simulink model "FinalProjectSimulation"  (R2023a)
settings: Solver=FixedStepAuto  StartTime=0.0  StopTime=t_final  FixedStep=dt  RelTol=1e-3
values from neighbouring files (symbols this model uses):
  dq_0 = [0; 0; 0]    [Initialization.m]
  dt = 1.00e-03    (= 0.001)    [Initialization.m]
  ikInitGuessSim = ikInitGuess    [defineTrajectory.m]
  P2_R2_waypoints = horzcat(initPosition,     [0.4000, 0, 0.8500 ... (first row only)    [defineTrajectory.m]
  P2_R2_waypointTimes = 0:3:6    [defineTrajectory.m]
  P2_R2_waypointVels = 0.1*[    1.5,  0,   1 ... (first row only)    [defineTrajectory.m]
  R2_T_R1 = [-1,  0,  0, P2_R1_pose(1)*2 + rod_length(1) ... (first row only)    [Initialization.m]
  rod_length = [0.20;0;0]    [Initialization.m]
  t_final = 30    [Initialization.m]
libraries: simulink x14, robotcorelib x6, robotmaniplib x1
settings Model: Creator=lukasz  LastModifiedBy=lukasz
settings OptimizationCC: ReuseModelBlockBuffer=off

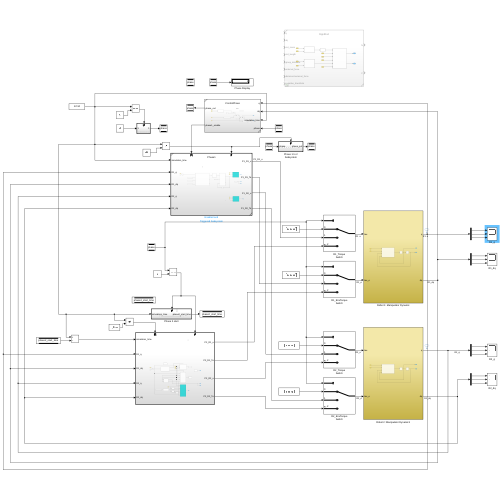
[thumbnail: Simulink's stored preview of the top-level diagram]
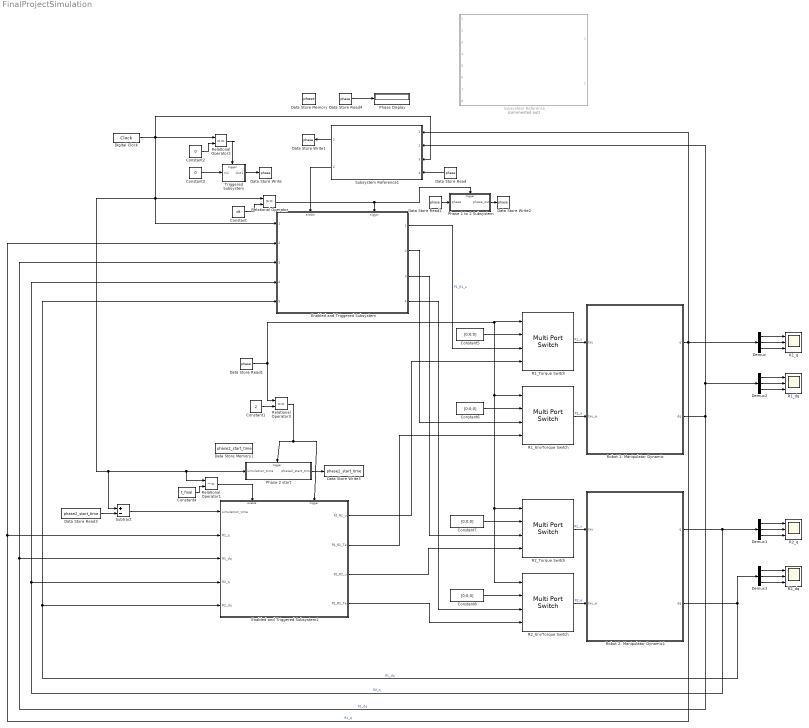
== system FinalProjectSimulation ==
  Constant : Constant  Value=dt
  Constant1 : Constant  Value=2
  Constant2 : Constant  Value=0
  Constant3 : Constant  Value=0  OutDataTypeStr=uint8
  Constant4 : Constant  Value=t_final
  Constant{5..8} (4 alike) : Constant  Value=[0;0;0]
  Data Store Memory : DataStoreMemory  DataStoreName=phase  WriteAfterWriteMsg=warning  ShowAdditionalParam=off  OutDataTypeStr=uint8
  Data Store Memory1 : DataStoreMemory  DataStoreName=phase2_start_time  WriteAfterWriteMsg=warning  InitialValue=-inf  ShowAdditionalParam=off
  Data Store Read{,1..2,4} (4 alike) : DataStoreRead  DataStoreName=phase  IndexOptions=Index vector (dialog)  Indices=1  OutputSizes=1
  Data Store Read3 : DataStoreRead  DataStoreName=phase2_start_time  IndexOptions=Index vector (dialog)  Indices=1  OutputSizes=1
  Data Store Write : DataStoreWrite  DataStoreName=phase  IndexOptions=Index vector (dialog)  Indices=1  OutputSizes=1
  Data Store Write1 : DataStoreWrite  DataStoreName=phase  IndexOptions=Index vector (dialog)  Indices=1  OutputSizes=1
  Data Store Write2 : DataStoreWrite  DataStoreName=phase  IndexOptions=Index vector (dialog)  Indices=1  OutputSizes=1
  Data Store Write3 : DataStoreWrite  DataStoreName=phase2_start_time  IndexOptions=Index vector (dialog)  Indices=1  OutputSizes=1
  Demux{,1..3} (4 alike) : Demux  Outputs=3
  Digital Clock : DigitalClock  SampleTime=dt
  Enabled and Triggered Subsystem : Subsystem  TreatAsAtomicUnit=on  ReferencedSubsystem=Phase1
  Enabled and Triggered Subsystem2 : Subsystem  TreatAsAtomicUnit=on
  Phase 1 to 2 Subsystem : Subsystem  TreatAsAtomicUnit=on
  Phase 2 start : Subsystem  TreatAsAtomicUnit=on
  Phase Display : Display
  R1_EnvTorque Switch : MultiPortSwitch  DataPortOrder=Specify indices  DataPortIndices={0,1,2}  SaturateOnIntegerOverflow=off  InputSameDT=off
  R1_Torque Switch : MultiPortSwitch  DataPortOrder=Specify indices  DataPortIndices={0,1,2}  SaturateOnIntegerOverflow=off  InputSameDT=off
  R1_dq : Scope  NumInputPorts=3
  R1_q : Scope  NumInputPorts=3
  R2_EnvTorque Switch : MultiPortSwitch  DataPortOrder=Specify indices  DataPortIndices={0,1,2}  SaturateOnIntegerOverflow=off  InputSameDT=off
  R2_Torque Switch : MultiPortSwitch  DataPortOrder=Specify indices  DataPortIndices={0,1,2}  SaturateOnIntegerOverflow=off  InputSameDT=off
  R2_dq : Scope  NumInputPorts=3
  R2_q : Scope  NumInputPorts=3
  Relational Operator : RelationalOperator  OutDataTypeStr=boolean  RndMeth=Simplest  InputSameDT=off
  Relational Operator1 : RelationalOperator  Operator=~=  OutDataTypeStr=boolean  RndMeth=Simplest  InputSameDT=off
  Relational Operator2 : RelationalOperator  Operator===  OutDataTypeStr=boolean  RndMeth=Simplest  InputSameDT=off
  Relational Operator3 : RelationalOperator  Operator===  OutDataTypeStr=boolean  RndMeth=Simplest  InputSameDT=off
  Robot 1: Manipulator Dynamic : Subsystem
  Robot 2: Manipulator Dynamic1 : Subsystem
  Subsystem Reference : Subsystem  Commented=on  ReferencedSubsystem=RigidRod
  Subsystem Reference1 : Subsystem  ReferencedSubsystem=ControlPhase
  Subtract : Sum  Inputs=+-
  Triggered Subsystem : Subsystem  TreatAsAtomicUnit=on
  wires:
  Demux/1 -> R1_q/1
  Demux/2 -> R1_q/2
  Demux/3 -> R1_q/3
  Constant/1 -> Relational Operator/2
  Relational Operator/1 -> Phase 1 to 2 Subsystem/Trigger, Enabled and Triggered Subsystem/Trigger
  Enabled and Triggered Subsystem/1 -> R1_Torque Switch/3  "P1_R1_u"
  R1_Torque Switch/1 -> Robot 1: Manipulator Dynamic/1(tau)  "R1_u"
  Robot 1: Manipulator Dynamic/2(dq) -> Subsystem Reference1/2, Demux2/1, Enabled and Triggered Subsystem/3, Enabled and Triggered Subsystem2/3(R1_dq)  "R1_dq"
  Robot 1: Manipulator Dynamic/1(q) -> Enabled and Triggered Subsystem/2, Enabled and Triggered Subsystem2/2(R1_q), Subsystem Reference1/1, Demux/1  "R1_q"
  Subsystem Reference1/2 -> Enabled and Triggered Subsystem/Enable
  Constant2/1 -> Relational Operator2/2
  Relational Operator2/1 -> Triggered Subsystem/Trigger
  Triggered Subsystem/1(Out1) -> Data Store Write/1
  Constant3/1 -> Triggered Subsystem/1(In1)
  Data Store Read/1 -> Subsystem Reference1/4
  Subsystem Reference1/1 -> Data Store Write1/1
  Data Store Read1/1 -> Relational Operator3/1, R1_Torque Switch/1, R2_EnvTorque Switch/1, R2_Torque Switch/1, R1_EnvTorque Switch/1
  Phase 1 to 2 Subsystem/1(phase_out) -> Data Store Write2/1
  Data Store Read2/1 -> Phase 1 to 2 Subsystem/1(phase)
  Constant1/1 -> Relational Operator3/2
  Relational Operator3/1 -> Enabled and Triggered Subsystem2/Trigger, Phase 2 start/Trigger
  Digital Clock/1 -> Relational Operator/1, Enabled and Triggered Subsystem/1, Relational Operator1/1, Phase 2 start/1(simulation_time), Subtract/1, Subsystem Reference1/3, Relational Operator2/1
  Data Store Read4/1 -> Phase Display/1
  Enabled and Triggered Subsystem/2 -> R1_EnvTorque Switch/3
  R1_EnvTorque Switch/1 -> Robot 1: Manipulator Dynamic/2(tau_e)  "R1_e"
  Enabled and Triggered Subsystem2/1(P2_R1_u) -> R1_Torque Switch/4
  Enabled and Triggered Subsystem2/2(P2_R1_Te) -> R1_EnvTorque Switch/4
  Phase 2 start/1(phase2_start_time) -> Data Store Write3/1
  Subtract/1 -> Enabled and Triggered Subsystem2/1(simulation_time)
  Data Store Read3/1 -> Subtract/2
  Relational Operator1/1 -> Enabled and Triggered Subsystem2/Enable
  Constant4/1 -> Relational Operator1/2
  R2_EnvTorque Switch/1 -> Robot 2: Manipulator Dynamic1/2(tau_e)  "R2_e"
  R2_Torque Switch/1 -> Robot 2: Manipulator Dynamic1/1(tau)  "R2_u"
  Demux1/3 -> R2_q/3
  Robot 2: Manipulator Dynamic1/1(q) -> Enabled and Triggered Subsystem/4, Enabled and Triggered Subsystem2/4(R2_q), Demux1/1  "R2_q"
  Demux1/1 -> R2_q/1
  Demux1/2 -> R2_q/2
  Enabled and Triggered Subsystem2/3(P2_R2_u) -> R2_Torque Switch/4
  Enabled and Triggered Subsystem2/4(P2_R2_Te) -> R2_EnvTorque Switch/4
  Enabled and Triggered Subsystem/3 -> R2_Torque Switch/3
  Enabled and Triggered Subsystem/4 -> R2_EnvTorque Switch/3
  Robot 2: Manipulator Dynamic1/2(dq) -> Enabled and Triggered Subsystem/5, Enabled and Triggered Subsystem2/5(R2_dq), Demux3/1  "R1_dq"
  Constant5/1 -> R1_Torque Switch/2
  Constant6/1 -> R1_EnvTorque Switch/2
  Constant7/1 -> R2_Torque Switch/2
  Constant8/1 -> R2_EnvTorque Switch/2
  Demux2/3 -> R1_dq/3
  Demux2/1 -> R1_dq/1
  Demux2/2 -> R1_dq/2
  Demux3/3 -> R2_dq/3
  Demux3/2 -> R2_dq/2
  Demux3/1 -> R2_dq/1

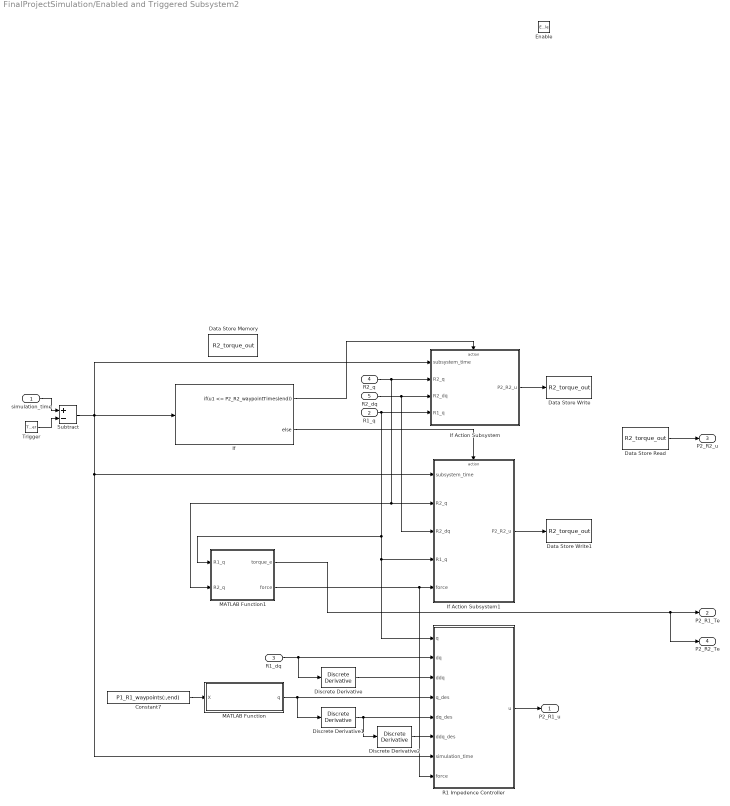
== system FinalProjectSimulation/Enabled and Triggered Subsystem2 ==
  simulation_time : Inport
  R1_q : Inport  Port=2
  R1_dq : Inport  Port=3
  R2_q : Inport  Port=4
  R2_dq : Inport  Port=5
  Enable : EnablePort
  Trigger : TriggerPort  VariantControl=(inherit)  ShowOutputPort=on
  Constant7 : Constant  Value=P1_R1_waypoints(:,end)  VectorParams1D=off  SampleTime=-1
  Data Store Memory : DataStoreMemory  DataStoreName=R2_torque_out  WriteAfterWriteMsg=warning  InitialValue=[0;0;0]  ShowAdditionalParam=off  Dimensions=3
  Data Store Read : DataStoreRead  DataStoreName=R2_torque_out  IndexOptions=Index vector (dialog)  Indices=1  OutputSizes=1
  Data Store Write : DataStoreWrite  DataStoreName=R2_torque_out  IndexOptions=Index vector (dialog)  Indices=1  OutputSizes=1
  Data Store Write1 : DataStoreWrite  DataStoreName=R2_torque_out  IndexOptions=Index vector (dialog)  Indices=1  OutputSizes=1
  Discrete Derivative : simulink/Discrete/Discrete Derivative  gainval=1.0  ICPrevScaledInput=1  OutMin=[]  OutMax=[]  OutDataType=fixdt(1, 16)  OutScaling=2^-10  DoSatur=off
  Discrete Derivative1 : simulink/Discrete/Discrete Derivative  gainval=1.0  ICPrevScaledInput=1  OutMin=[]  OutMax=[]  OutDataType=fixdt(1, 16)  OutScaling=2^-10  DoSatur=off
  Discrete Derivative2 : simulink/Discrete/Discrete Derivative  gainval=1.0  ICPrevScaledInput=1  OutMin=[]  OutMax=[]  OutDataType=fixdt(1, 16)  OutScaling=2^-10  DoSatur=off
  If : If  IfExpression=u1 <= P2_R2_waypointTimes(end)
  If Action Subsystem : Subsystem  TreatAsAtomicUnit=on
  If Action Subsystem1 : Subsystem  TreatAsAtomicUnit=on
  MATLAB Function : MATLAB Function  TreatAsAtomicUnit=on
  MATLAB Function1 : MATLAB Function  TreatAsAtomicUnit=on
  R1 Impedence Controller : Subsystem
  Subtract : Sum  Inputs=+-
  P2_R1_u : Outport
  P2_R1_Te : Outport  Port=2
  P2_R2_u : Outport  Port=3
  P2_R2_Te : Outport  Port=4
  wires:
  R2_dq/1 -> If Action Subsystem1/3(R2_dq), If Action Subsystem/3(R2_dq)
  R1 Impedence Controller/1(u) -> P2_R1_u/1
  Trigger/1 -> Subtract/2
  R2_q/1 -> MATLAB Function1/2(R2_q), If Action Subsystem1/2(R2_q), If Action Subsystem/2(R2_q)
  simulation_time/1 -> Subtract/1
  MATLAB Function1/1(torque_e) -> P2_R2_Te/1, P2_R1_Te/1
  R1_dq/1 -> Discrete Derivative/1, R1 Impedence Controller/2(dq)
  Constant7/1 -> MATLAB Function/1(X)
  MATLAB Function/1(q) -> Discrete Derivative1/1, R1 Impedence Controller/4(q_des)
  If/1 -> If Action Subsystem/Action
  Subtract/1 -> If/1, If Action Subsystem/1(subsystem_time), R1 Impedence Controller/7(simulation_time), If Action Subsystem1/1(subsystem_time)
  If Action Subsystem/1(P2_R2_u) -> Data Store Write/1
  Data Store Read/1 -> P2_R2_u/1
  If/2 -> If Action Subsystem1/Action
  If Action Subsystem1/1(P2_R2_u) -> Data Store Write1/1
  R1_q/1 -> If Action Subsystem/4(R1_q), If Action Subsystem1/4(R1_q), R1 Impedence Controller/1(q), MATLAB Function1/1(R1_q)
  Discrete Derivative/1 -> R1 Impedence Controller/3(ddq)
  Discrete Derivative1/1 -> Discrete Derivative2/1, R1 Impedence Controller/5(dq_des)
  Discrete Derivative2/1 -> R1 Impedence Controller/6(ddq_des)
  MATLAB Function1/2(force) -> R1 Impedence Controller/8(force), If Action Subsystem1/5(force)

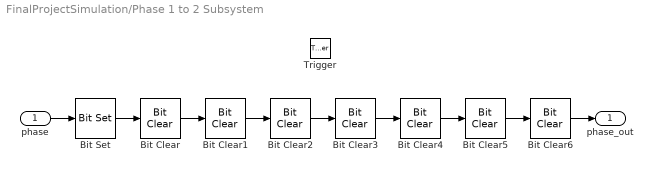
== system FinalProjectSimulation/Phase 1 to 2 Subsystem ==
  phase : Inport
  Trigger : TriggerPort  VariantControl=(inherit)
  Bit Clear : simulink/Logic and Bit Operations/Bit Clear  iBit=1
  Bit Clear1 : simulink/Logic and Bit Operations/Bit Clear  iBit=2
  Bit Clear2 : simulink/Logic and Bit Operations/Bit Clear  iBit=3
  Bit Clear3 : simulink/Logic and Bit Operations/Bit Clear  iBit=4
  Bit Clear4 : simulink/Logic and Bit Operations/Bit Clear  iBit=5
  Bit Clear5 : simulink/Logic and Bit Operations/Bit Clear  iBit=6
  Bit Clear6 : simulink/Logic and Bit Operations/Bit Clear  iBit=7
  Bit Set : simulink/Logic and Bit Operations/Bit Set  iBit=0
  phase_out : Outport
  wires:
  Bit Clear6/1 -> phase_out/1
  Bit Clear5/1 -> Bit Clear6/1
  Bit Clear4/1 -> Bit Clear5/1
  Bit Clear3/1 -> Bit Clear4/1
  Bit Clear2/1 -> Bit Clear3/1
  Bit Clear1/1 -> Bit Clear2/1
  Bit Clear/1 -> Bit Clear1/1
  phase/1 -> Bit Set/1
  Bit Set/1 -> Bit Clear/1

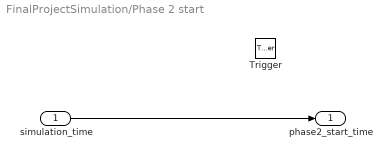
== system FinalProjectSimulation/Phase 2 start ==
  simulation_time : Inport
  Trigger : TriggerPort  VariantControl=(inherit)
  phase2_start_time : Outport
  wires:
  simulation_time/1 -> phase2_start_time/1

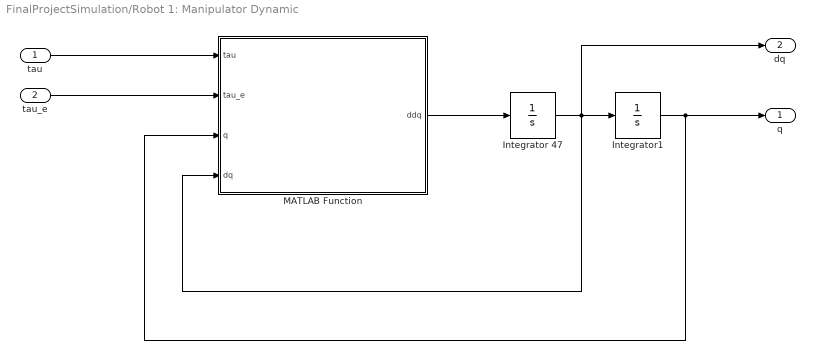
== system FinalProjectSimulation/Robot 1: Manipulator Dynamic ==
  tau : Inport
  tau_e : Inport  Port=2
  Integrator 47 : Integrator  InitialCondition=dq_0
  Integrator1 : Integrator  InitialCondition=ikInitGuessSim
  MATLAB Function : MATLAB Function  TreatAsAtomicUnit=on
  q : Outport
  dq : Outport  Port=2
  wires:
  MATLAB Function/1(ddq) -> Integrator 47/1
  tau/1 -> MATLAB Function/1(tau)
  tau_e/1 -> MATLAB Function/2(tau_e)
  Integrator1/1 -> q/1, MATLAB Function/3(q)
  Integrator 47/1 -> dq/1, MATLAB Function/4(dq), Integrator1/1

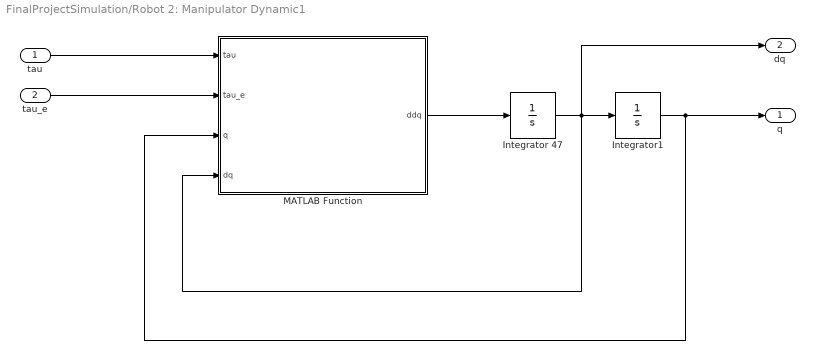
== system FinalProjectSimulation/Robot 2: Manipulator Dynamic1 ==
  tau : Inport
  tau_e : Inport  Port=2
  Integrator 47 : Integrator  InitialCondition=dq_0
  Integrator1 : Integrator  InitialCondition=ikInitGuessSim
  MATLAB Function : MATLAB Function  TreatAsAtomicUnit=on
  q : Outport
  dq : Outport  Port=2
  wires:
  MATLAB Function/1(ddq) -> Integrator 47/1
  tau/1 -> MATLAB Function/1(tau)
  tau_e/1 -> MATLAB Function/2(tau_e)
  Integrator1/1 -> q/1, MATLAB Function/3(q)
  Integrator 47/1 -> dq/1, MATLAB Function/4(dq), Integrator1/1

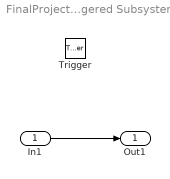
== system FinalProjectSimulation/Triggered Subsystem ==
  In1 : Inport
  Trigger : TriggerPort  VariantControl=(inherit)
  Out1 : Outport
  wires:
  In1/1 -> Out1/1

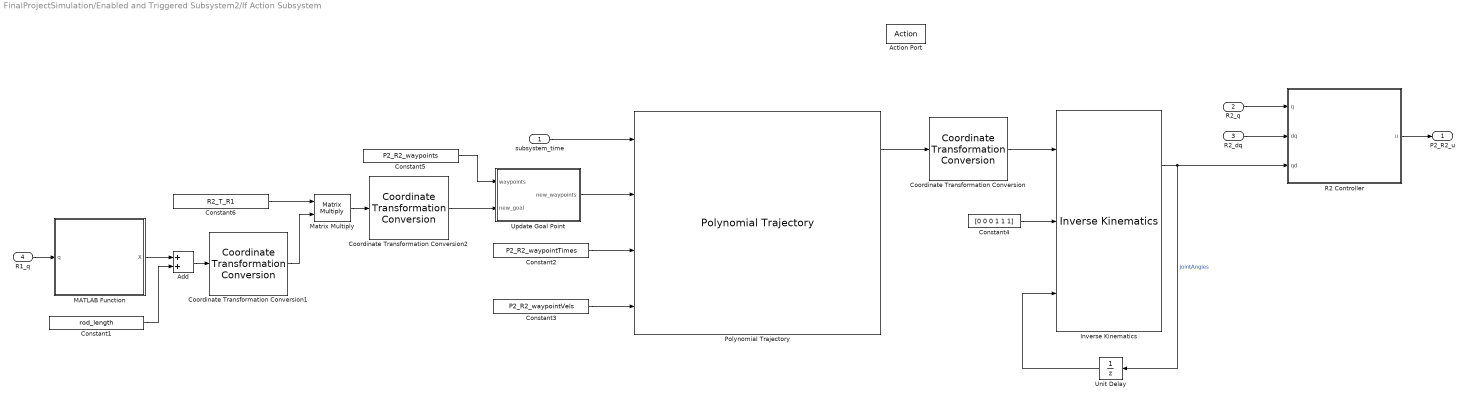
== system FinalProjectSimulation/Enabled and Triggered Subsystem2/If Action Subsystem ==
  subsystem_time : Inport
  R2_q : Inport  Port=2
  R2_dq : Inport  Port=3
  R1_q : Inport  Port=4
  Action Port : ActionPort  ActionPortLabel=if(u1 <= P2_R2_waypointTimes(end))
  Add : Sum
  Constant1 : Constant  Value=rod_length  VectorParams1D=off  SampleTime=-1
  Constant2 : Constant  Value=P2_R2_waypointTimes  VectorParams1D=off  SampleTime=-1
  Constant3 : Constant  Value=P2_R2_waypointVels  VectorParams1D=off  SampleTime=-1
  Constant4 : Constant  Value=[0 0 0 1 1 1]  VectorParams1D=off
  Constant5 : Constant  Value=P2_R2_waypoints  VectorParams1D=off  SampleTime=-1
  Constant6 : Constant  Value=R2_T_R1  VectorParams1D=off  SampleTime=-1
  Coordinate Transformation Conversion : robotcorelib/Coordinate Transformation Conversion  InputRepresentation=Translation Vector  InputEulerSequence=ZYX  ShowTrVecInputPort=on  OutputRepresentation=Homogeneous Transformation  OutputEulerSequence=ZYX  ShowTrVecOutputPort=on  SimulateUsing=Code generation
  Coordinate Transformation Conversion1 : robotcorelib/Coordinate Transformation Conversion  InputRepresentation=Translation Vector  InputEulerSequence=ZYX  ShowTrVecInputPort=on  OutputRepresentation=Homogeneous Transformation  OutputEulerSequence=ZYX  ShowTrVecOutputPort=on  SimulateUsing=Code generation
  Coordinate Transformation Conversion2 : robotcorelib/Coordinate Transformation Conversion  InputRepresentation=Homogeneous Transformation  InputEulerSequence=ZYX  ShowTrVecInputPort=on  OutputRepresentation=Translation Vector  OutputEulerSequence=ZYX  ShowTrVecOutputPort=on  SimulateUsing=Code generation
  Inverse Kinematics : robotmaniplib/Inverse Kinematics  RigidBodyTree=robot1  EndEffector=Link_EE  ShowInfo=on  SolverName=BFGS Gradient Projection  EnforceJointLimits=on  MaxIterations=1500  MaxTime=10  GradientTolerance=1e-7  SolutionTolerance=1e-6  StepTolerance=1e-14  ErrorChangeTolerance=1e-12  UseErrorDamping=on  DampingBias=0.0025  SimulateUsing=Code generation
  MATLAB Function : MATLAB Function  TreatAsAtomicUnit=on
  Matrix Multiply : Product  Multiplication=Matrix(*)  RndMeth=Round
  Polynomial Trajectory : robotcorelib/Polynomial Trajectory  WaypointSource=External  Waypoints=[ 0, 2, 1, 5, 0; -1, 3, 1, 4, 4 ]  TimePoints=[ 0, 1, 2, 3, 4 ]  TimeInterval=[ 1, 4 ]  Method=Cubic Polynomial  ParameterSource=External  VelocityBoundaryCondition=zeros( 2, 5 )  AccelerationBoundaryCondition=zeros( 2, 5 )  SimulateUsing=Interpreted execution
  R2 Controller : Subsystem
  Unit Delay : UnitDelay  InitialCondition=ikInitGuessSim  SampleTime=-1  HasFrameUpgradeWarning=on
  Update Goal Point : MATLAB Function  TreatAsAtomicUnit=on
  P2_R2_u : Outport
  wires:
  Update Goal Point/1(new_waypoints) -> Polynomial Trajectory/2
  Inverse Kinematics/1 -> R2 Controller/3(qd), Unit Delay/1  "jointAngles"
  Unit Delay/1 -> Inverse Kinematics/3
  subsystem_time/1 -> Polynomial Trajectory/1
  Constant3/1 -> Polynomial Trajectory/4
  Coordinate Transformation Conversion/1 -> Inverse Kinematics/1
  Constant4/1 -> Inverse Kinematics/2
  Polynomial Trajectory/1 -> Coordinate Transformation Conversion/1
  Constant2/1 -> Polynomial Trajectory/3
  R2_dq/1 -> R2 Controller/2(dq)
  R2_q/1 -> R2 Controller/1(q)
  R2 Controller/1(u) -> P2_R2_u/1
  R1_q/1 -> MATLAB Function/1(q)
  Coordinate Transformation Conversion2/1 -> Update Goal Point/2(new_goal)
  Constant5/1 -> Update Goal Point/1(waypoints)
  MATLAB Function/1(X) -> Add/1
  Add/1 -> Coordinate Transformation Conversion1/1
  Coordinate Transformation Conversion1/1 -> Matrix Multiply/2
  Matrix Multiply/1 -> Coordinate Transformation Conversion2/1
  Constant6/1 -> Matrix Multiply/1
  Constant1/1 -> Add/2

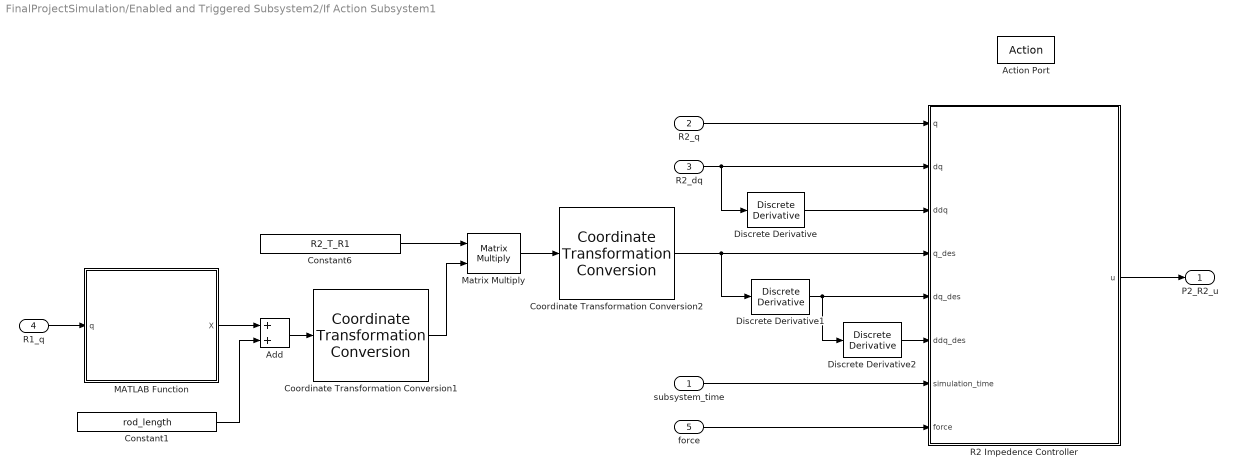
== system FinalProjectSimulation/Enabled and Triggered Subsystem2/If Action Subsystem1 ==
  subsystem_time : Inport
  R2_q : Inport  Port=2
  R2_dq : Inport  Port=3
  R1_q : Inport  Port=4
  force : Inport  Port=5
  Action Port : ActionPort  ActionPortLabel=else
  Add : Sum
  Constant1 : Constant  Value=rod_length  VectorParams1D=off  SampleTime=-1
  Constant6 : Constant  Value=R2_T_R1  VectorParams1D=off  SampleTime=-1
  Coordinate Transformation Conversion1 : robotcorelib/Coordinate Transformation Conversion  InputRepresentation=Translation Vector  InputEulerSequence=ZYX  ShowTrVecInputPort=on  OutputRepresentation=Homogeneous Transformation  OutputEulerSequence=ZYX  ShowTrVecOutputPort=on  SimulateUsing=Code generation
  Coordinate Transformation Conversion2 : robotcorelib/Coordinate Transformation Conversion  InputRepresentation=Homogeneous Transformation  InputEulerSequence=ZYX  ShowTrVecInputPort=on  OutputRepresentation=Translation Vector  OutputEulerSequence=ZYX  ShowTrVecOutputPort=on  SimulateUsing=Code generation
  Discrete Derivative : simulink/Discrete/Discrete Derivative  gainval=1.0  ICPrevScaledInput=1  OutMin=[]  OutMax=[]  OutDataType=fixdt(1, 16)  OutScaling=2^-10  DoSatur=off
  Discrete Derivative1 : simulink/Discrete/Discrete Derivative  gainval=1.0  ICPrevScaledInput=1  OutMin=[]  OutMax=[]  OutDataType=fixdt(1, 16)  OutScaling=2^-10  DoSatur=off
  Discrete Derivative2 : simulink/Discrete/Discrete Derivative  gainval=1.0  ICPrevScaledInput=1  OutMin=[]  OutMax=[]  OutDataType=fixdt(1, 16)  OutScaling=2^-10  DoSatur=off
  MATLAB Function : MATLAB Function  TreatAsAtomicUnit=on
  Matrix Multiply : Product  Multiplication=Matrix(*)  RndMeth=Round
  R2 Impedence Controller : Subsystem
  P2_R2_u : Outport
  wires:
  R2 Impedence Controller/1(u) -> P2_R2_u/1
  R2_dq/1 -> Discrete Derivative/1, R2 Impedence Controller/2(dq)
  R2_q/1 -> R2 Impedence Controller/1(q)
  subsystem_time/1 -> R2 Impedence Controller/7(simulation_time)
  R1_q/1 -> MATLAB Function/1(q)
  Coordinate Transformation Conversion1/1 -> Matrix Multiply/2
  Add/1 -> Coordinate Transformation Conversion1/1
  Constant1/1 -> Add/2
  MATLAB Function/1(X) -> Add/1
  Constant6/1 -> Matrix Multiply/1
  Matrix Multiply/1 -> Coordinate Transformation Conversion2/1
  Coordinate Transformation Conversion2/1 -> Discrete Derivative1/1, R2 Impedence Controller/4(q_des)
  Discrete Derivative/1 -> R2 Impedence Controller/3(ddq)
  Discrete Derivative1/1 -> Discrete Derivative2/1, R2 Impedence Controller/5(dq_des)
  Discrete Derivative2/1 -> R2 Impedence Controller/6(ddq_des)
  force/1 -> R2 Impedence Controller/8(force)

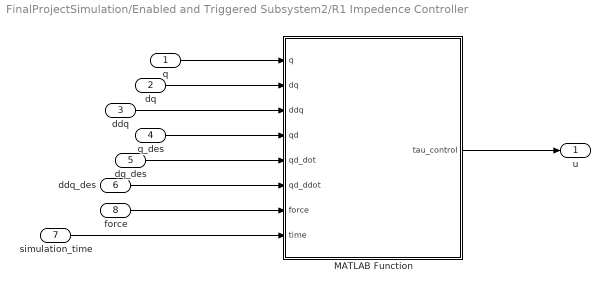
== system FinalProjectSimulation/Enabled and Triggered Subsystem2/R1 Impedence Controller ==
  q : Inport
  dq : Inport  Port=2
  ddq : Inport  Port=3
  q_des : Inport  Port=4
  dq_des : Inport  Port=5
  ddq_des : Inport  Port=6
  simulation_time : Inport  Port=7
  force : Inport  Port=8
  MATLAB Function : MATLAB Function  TreatAsAtomicUnit=on
  u : Outport
  wires:
  dq/1 -> MATLAB Function/2(dq)
  MATLAB Function/1(tau_control) -> u/1
  q_des/1 -> MATLAB Function/4(qd)
  q/1 -> MATLAB Function/1(q)
  ddq_des/1 -> MATLAB Function/6(qd_ddot)
  dq_des/1 -> MATLAB Function/5(qd_dot)
  simulation_time/1 -> MATLAB Function/8(time)
  ddq/1 -> MATLAB Function/3(ddq)
  force/1 -> MATLAB Function/7(force)

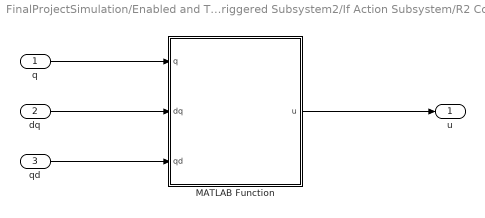
== system FinalProjectSimulation/Enabled and Triggered Subsystem2/If Action Subsystem/R2 Controller ==
  q : Inport
  dq : Inport  Port=2
  qd : Inport  Port=3
  MATLAB Function : MATLAB Function  TreatAsAtomicUnit=on
  u : Outport
  wires:
  q/1 -> MATLAB Function/1(q)
  qd/1 -> MATLAB Function/3(qd)
  MATLAB Function/1(u) -> u/1
  dq/1 -> MATLAB Function/2(dq)

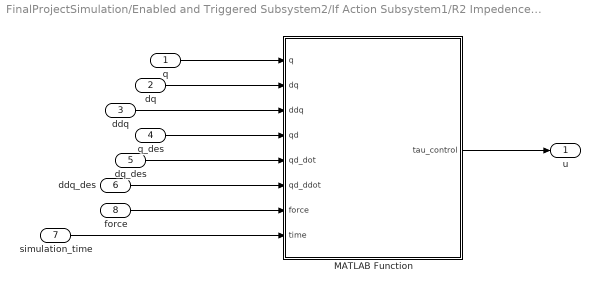
== system FinalProjectSimulation/Enabled and Triggered Subsystem2/If Action Subsystem1/R2 Impedence Controller ==
  q : Inport
  dq : Inport  Port=2
  ddq : Inport  Port=3
  q_des : Inport  Port=4
  dq_des : Inport  Port=5
  ddq_des : Inport  Port=6
  simulation_time : Inport  Port=7
  force : Inport  Port=8
  MATLAB Function : MATLAB Function  TreatAsAtomicUnit=on
  u : Outport
  wires:
  dq/1 -> MATLAB Function/2(dq)
  MATLAB Function/1(tau_control) -> u/1
  q_des/1 -> MATLAB Function/4(qd)
  q/1 -> MATLAB Function/1(q)
  ddq_des/1 -> MATLAB Function/6(qd_ddot)
  dq_des/1 -> MATLAB Function/5(qd_dot)
  simulation_time/1 -> MATLAB Function/8(time)
  ddq/1 -> MATLAB Function/3(ddq)
  force/1 -> MATLAB Function/7(force)

== matlab function FinalProjectSimulation/Enabled and Triggered Subsystem2/If Action Subsystem1/MATLAB Function ==
  data: q input; X output
function X = FWDKinematics(q)
%%% Forward Kinematic Function


%% Joint Space variables
% q is 3*1 vector of joint variables (radian), q = [q1;q2;q3]
q1 = q(1);
q2 = q(2);
q3 = q(3);

%% general physical parameters
l1 = 0.6731;
l2 = 0.432;
l3 = 0.434;
lc2 = 0.216;
lc3 = 0.164;

%% Forward Kinematic
% X is 3*1 vecto of end-effector position in task space, X = [x;y;z]

x = cos(q1) * (l2 * cos(q2) + l3 * sin(q2 + q3));
y = sin(q1) * (l2 * cos(q2) + l3 * sin(q2 + q3));
z = l1 - l2 * sin(q2) + l3 * cos(q2 + q3);

X = [x;y;z]

== matlab function FinalProjectSimulation/Enabled and Triggered Subsystem2/MATLAB Function1 ==
  data: R1_q input; torque_e output; R2_q input; force output
function [torque_e, force] = fcn(R1_q, R2_q)

k = [1, 0, 0;
      0, 1, 0;
      0, 0, 1];
comp = [0;0;0];
force = k * comp;
torque_e = [0;0;0];

== matlab function FinalProjectSimulation/Robot 1: Manipulator Dynamic/MATLAB Function ==
  data: tau input; tau_e input; q input; ddq output; dq input
function ddq = DynamicModel( tau, tau_e, q, dq)
%%%%%
% 3-DOF Puma-560 Dynamic Model Function
% H(q)* ddq + C(q) * dq + G = tau + tau_e
% q is 3*1 vector of joint variables (radian)
% H(q) is the inertia matrix
% C(q) is the matrix of Coriolis and centrifugal forces
% G(q) is  the vector of potential forces Parameters
% tau is control torque 
% tau_e is the external torque due to the interaction with the environment
%%%%%

%% Joint Space variables

q1 = q(1);
q2 = q(2);
q3 = q(3);

dq1 = dq(1);
dq2 = dq(2);
dq3 = dq(3);

%% general physical parameters

l1 = 0.6731;
l2 = 0.432;
l3 = 0.434;
lc2 = 0.216;
lc3 = 0.164;
m2 = 15.46;
m3 = 9.55;
J = 0.302;

%% Inertia Matrix Parameters

J1 = m3 * lc3^2;
J12 = (m2 * lc2^2) + (m3 * l2^2);
J13 = l2 * lc3 * m3;


h11 = J + J1 * (sin(q2 + q3))^2 + J12 * (cos(q2))^2 + 2 * J13 * cos(q2) * sin(q2+q3);
h22 = J1 + J12 + 2 * J13 * sin(q3);
h23 = J1 + J13 * sin(q3);
h32 = h23;
h33 = J1;

H = [h11, 0 ,0 ;
    0 , h22, h23;
    0 , h32, h33];

%% Coriolis Matrix Parameters

c12_1 = J1 * sin(2 * (q1 + q2)) - J12 * sin(2 * q2) + 2 * J13 * cos(2 * q2 +q3);
c13_1 = J1 * sin(2 * (q2 + q3)) + 2 * J13 * cos(q2) * cos(q2 + q3);
c11_2 = (1/2) * (-J1 * sin(2 * (q2 + q3)) + J12 * sin(2 * q2) - 2 * J13 * cos(2 * q2 + q3));
c22_2 = 2 * J13 * cos(q3);
c23_2 = J13 * cos(q3);
c22_3 = -J13 * cos(q3) * dq2;
c11_3 = (-1/2) * (J1 * sin(2 * (q2 + q3)) + J13 * cos(q2) * cos(q2 + q3));

C = [0, c12_1 * dq1, c13_1 * dq3;
    c11_2 * dq1, 0 , c22_2 * dq2 + c23_2 * dq3;
    c11_3 * dq1, c22_3 * dq2, 0];

%% Vector of Potential Forces Parameters

g = 9.81;

g21 = -g * (lc3 * m3 * sin(q2 + q3) + lc2 * m2 * cos(q2) + l2 * m3 * cos(q2));
g31 = -g * (lc3 * m3 * sin(q2 + q3));

G = [0;
    g21;
    g31];

%% Function output

ddq = inv(H)*(tau + tau_e - C * dq - G);

== matlab function FinalProjectSimulation/Robot 2: Manipulator Dynamic1/MATLAB Function ==
  data: tau input; tau_e input; q input; ddq output; dq input
function ddq = DynamicModel( tau, tau_e, q, dq)
%%%%%
% 3-DOF Puma-560 Dynamic Model Function
% H(q)* ddq + C(q) * dq + G = tau + tau_e
% q is 3*1 vector of joint variables (radian)
% H(q) is the inertia matrix
% C(q) is the matrix of Coriolis and centrifugal forces
% G(q) is  the vector of potential forces Parameters
% tau is control torque 
% tau_e is the external torque due to the interaction with the environment
%%%%%

%% Joint Space variables

q1 = q(1);
q2 = q(2);
q3 = q(3);

dq1 = dq(1);
dq2 = dq(2);
dq3 = dq(3);

%% general physical parameters

l1 = 0.6731;
l2 = 0.432;
l3 = 0.434;
lc2 = 0.216;
lc3 = 0.164;
m2 = 15.46;
m3 = 9.55;
J = 0.302;

%% Inertia Matrix Parameters

J1 = m3 * lc3^2;
J12 = (m2 * lc2^2) + (m3 * l2^2);
J13 = l2 * lc3 * m3;


h11 = J + J1 * (sin(q2 + q3))^2 + J12 * (cos(q2))^2 + 2 * J13 * cos(q2) * sin(q2+q3);
h22 = J1 + J12 + 2 * J13 * sin(q3);
h23 = J1 + J13 * sin(q3);
h32 = h23;
h33 = J1;

H = [h11, 0 ,0 ;
    0 , h22, h23;
    0 , h32, h33];

%% Coriolis Matrix Parameters

c12_1 = J1 * sin(2 * (q1 + q2)) - J12 * sin(2 * q2) + 2 * J13 * cos(2 * q2 +q3);
c13_1 = J1 * sin(2 * (q2 + q3)) + 2 * J13 * cos(q2) * cos(q2 + q3);
c11_2 = (1/2) * (-J1 * sin(2 * (q2 + q3)) + J12 * sin(2 * q2) - 2 * J13 * cos(2 * q2 + q3));
c22_2 = 2 * J13 * cos(q3);
c23_2 = J13 * cos(q3);
c22_3 = -J13 * cos(q3) * dq2;
c11_3 = (-1/2) * (J1 * sin(2 * (q2 + q3)) + J13 * cos(q2) * cos(q2 + q3));

C = [0, c12_1 * dq1, c13_1 * dq3;
    c11_2 * dq1, 0 , c22_2 * dq2 + c23_2 * dq3;
    c11_3 * dq1, c22_3 * dq2, 0];

%% Vector of Potential Forces Parameters

g = 9.81;

g21 = -g * (lc3 * m3 * sin(q2 + q3) + lc2 * m2 * cos(q2) + l2 * m3 * cos(q2));
g31 = -g * (lc3 * m3 * sin(q2 + q3));

G = [0;
    g21;
    g31];

%% Function output

ddq = inv(H)*(tau + tau_e - C * dq - G);

== matlab function FinalProjectSimulation/Enabled and Triggered Subsystem2/R1 Impedence Controller/MATLAB Function ==
  data: q input; dq input; ddq input; tau_control output; qd input; qd_dot input; qd_ddot input; force input; time input
function tau_control   = fcn(q, dq, ddq, qd, qd_dot, qd_ddot,force,...
                                                                  time)
% reset first qd_ddot
if (time < 0.003)
    qd_ddot = [0;0;0];
    qd_dot = [0;0;0];
    ddq = [0;0;0];
end


%% Joint Space variables

q1 = q(1);
q2 = q(2);
q3 = q(3);

dq1 = dq(1);
dq2 = dq(2);
dq3 = dq(3);

%% general physical parameters

l1 = 0.6731;
l2 = 0.432;
l3 = 0.434;
lc2 = 0.216;
lc3 = 0.164;
m2 = 15.46;
m3 = 9.55;
J = 0.302;

%% Inertia Matrix Parameters

J1 = m3 * lc3^2;
J12 = (m2 * lc2^2) + (m3 * l2^2);
J13 = l2 * lc3 * m3;


h11 = J + J1 * (sin(q2 + q3))^2 + J12 * (cos(q2))^2 + 2 * J13 * cos(q2) * sin(q2+q3);
h22 = J1 + J12 + 2 * J13 * sin(q3);
h23 = J1 + J13 * sin(q3);
h32 = h23;
h33 = J1;

H = [h11, 0 ,0 ;
    0 , h22, h23;
    0 , h32, h33];

%% Coriolis Matrix Parameters

c12_1 = J1 * sin(2 * (q1 + q2)) - J12 * sin(2 * q2) + 2 * J13 * cos(2 * q2 +q3);
c13_1 = J1 * sin(2 * (q2 + q3)) + 2 * J13 * cos(q2) * cos(q2 + q3);
c11_2 = (1/2) * (-J1 * sin(2 * (q2 + q3)) + J12 * sin(2 * q2) - 2 * J13 * cos(2 * q2 + q3));
c22_2 = 2 * J13 * cos(q3);
c23_2 = J13 * cos(q3);
c22_3 = -J13 * cos(q3) * dq2;
c11_3 = (-1/2) * (J1 * sin(2 * (q2 + q3)) + J13 * cos(q2) * cos(q2 + q3));

C = [0, c12_1 * dq1, c13_1 * dq3;
    c11_2 * dq1, 0 , c22_2 * dq2 + c23_2 * dq3;
    c11_3 * dq1, c22_3 * dq2, 0];

%% Vector of Potential Forces Parameters

g = 9.81;

g21 = -g * (lc3 * m3 * sin(q2 + q3) + lc2 * m2 * cos(q2) + l2 * m3 * cos(q2));
g31 = -g * (lc3 * m3 * sin(q2 + q3));

G = [0;
    g21;
    g31];


%% get Jacobians
J = jacobian(q);
dJ = dJacobian(q,dq);

%% convert to task space
Hp = inv(J') * H * inv(J);
Cp = inv(J') * C * inv(J) - Hp * dJ * inv(J);
Gp = inv(J') * G;

%% desired behaviour 
Hm = [1 0 0; 0 1 0; 0 0 1];
Dm = [20 0 0; 0 20 0; 0 0 20];
Km = [500 0 0; 0 500  0; 0 0 500];

%% get postion and its derivs
p = fwdKin(q);
dp = J * dq;
ddp = dJ * dq + J * ddq;

%% get desired postion and its derivs
pd = fwdKin(qd);
pd_dot = jacobian(qd) * qd_dot;
pd_ddot = dJacobian(qd,qd_dot) * qd_dot + jacobian(qd) * qd_ddot;

%% define u note

u_note = pd_ddot + inv(Hm) * (Dm * (pd_dot-dp) + Km*(pd - p) + force);
inv_hm = inv(Hm);
%% define tau_control

tau_control = J' * (Hp * u_note + Cp * dp + Gp - force);


function [X] = fwdKin(Q)
    s1 = sin(Q(1, :));
    c1 = cos(Q(1, :));
    s2 = sin(Q(2, :));
    c2 = cos(Q(2, :));
    s23 = sin(Q(2, :) + Q(3, :));
    c23 = cos(Q(2, :) + Q(3, :));
    l = [0.6731; 0.432; 0.434];
    
    X = zeros(3,1);
    X(1, :) = c1.*(l(2)*c2 + l(3)*s23);
    X(2, :) = s1.*(l(2)*c2 + l(3)*s23);
    X(3, :) = l(1) - l(2)*s2 + l(3)*c23;

function dJ = dJacobian(Q, dQ)
    l = [0.6731; 0.432; 0.434];
    s1 = sin(Q(1));
    c1 = cos(Q(1));
    s2 = sin(Q(2));
    c2 = cos(Q(2));
    s23 = sin(Q(2) + Q(3));
    c23 = cos(Q(2) + Q(3));

    % dJi derivative of each element of Jacobian wrt i-th variable            
    %--- 1 ---
    dJ1 = [-c1*(l(2)*c2 + l(3)*s23), -s1*(-l(2)*s2 + l(3)*c23), -l(3)*s1*c23;...
           -s1*(l(2)*c2 + l(3)*s23),  c1*(-l(2)*s2 + l(3)*c23),  l(3)*c1*c23;...
           0, 0, 0];
    %--- 2 ---   
    dJ2 = [-s1*(-l(2)*s2 + l(3)*c23), -c1*(l(2)*c2 + l(3)*s23), -l(3)*c1*s23;...
            c1*(-l(2)*s2 + l(3)*c23), -s1*(l(2)*c2 + l(3)*s23), -l(3)*s1*s23;...
            0, l(2)*s2 - l(3)*c23, -l(3)*c23];

    %--- 3 ---
    dJ3 = -l(3)*[ s1*c23, c1*s23, c1*s23;...
                 -c1*c23, s1*s23, s1*s23;...
                 0, c23, c23];
    %--- dJ ---
    dJ = dJ1*dQ(1) + dJ2*dQ(2) + dJ3*dQ(3);

function [J] = jacobian(q)

l = [0.6731; 0.432; 0.434];
s1 = sin(q(1));
c1 = cos(q(1));
s2 = sin(q(2));
c2 = cos(q(2));
s23 = sin(q(2) + q(3));
c23 = cos(q(2) + q(3));

J = zeros(3,3);

J(1, 1) = -s1*( l(2)*c2 + l(3)*s23);
J(1, 2) =  c1*(-l(2)*s2 + l(3)*c23);
J(1, 3) = l(3)*c1*c23;

J(2, 1) = c1*( l(2)*c2 + l(3)*s23);
J(2, 2) = s1*(-l(2)*s2 + l(3)*c23);
J(2, 3) = l(3)*s1*c23;

J(3, 2) = -l(2)*c2 - l(3)*s23;
J(3, 3) = -l(3)*s23;

== matlab function FinalProjectSimulation/Enabled and Triggered Subsystem2/If Action Subsystem/R2 Controller/MATLAB Function ==
  data: q input; dq input; u output; qd input
function u = fcn(q, dq, qd)
% PD + gravity compensation controller function

%% general physical parameters

l1 = 0.6731;
l2 = 0.432;
l3 = 0.434;
lc2 = 0.216;
lc3 = 0.164;
m2 = 15.46;
m3 = 9.55;
J = 0.302;

%% Joint Space variables

q1 = q(1);
q2 = q(2);
q3 = q(3);

dq1 = dq(1);
dq2 = dq(2);
dq3 = dq(3);
g = 9.81;

%% Vector of Potential Forces Parameters

g21 = -g * (lc3 * m3 * sin(q2 + q3) + lc2 * m2 * cos(q2) + l2 * m3 * cos(q2));
g31 = -g * (lc3 * m3 * sin(q2 + q3));

G = [0;
    g21;
    g31];

%% PD Controller Parameters 

Kp = [10,0,0; 0, 10 ,0; 0, 0 , 10];  %  Kp is 3*3 matrix of proportional gain 
Kd = [1,0,0; 0, 1 ,0; 0, 0 , 1]; %Kd is 3*3 matrix of derivative gain

%% Control law

u = - Kp * (q - qd) - Kd * dq + G;

== matlab function FinalProjectSimulation/Enabled and Triggered Subsystem2/MATLAB Function ==
  data: X input; q output
function q = INVKinematics(X)
%%% Inverse Kinematic Function
% X is 3*1 vecto of end-effector position in task space, X = [x;y;z]
x = X(1);
y = X(2);
z = X(3);

%% general physical parameters
l1 = 0.6731;
l2 = 0.432;
l3 = 0.434;
lc2 = 0.216;
lc3 = 0.164;

r = sqrt(x^2 + y^2);
R = sqrt(r^2 + (z-l1)^2);
a = atan2(r, z-l1);

%% Inverse Kinematics
% q is 3*1 vector of joint variables (radian), q = [q1;q2;q3]
q1 = atan2(y,x);
q2 = a - atan2(R^2 + l2^2 -l3^2,sqrt(((l2 + l3)^2 - R^2) * (R^2 - (l2 - l3)^2)));
q3 = atan2(R^2 - (l2^2 + l3^2) , sqrt(((l2 + l3)^2 - R^2) * (R^2 - (l2 - l3)^2)));

q = [q1;q2;q3]

== matlab function FinalProjectSimulation/Enabled and Triggered Subsystem2/If Action Subsystem1/R2 Impedence Controller/MATLAB Function ==
  data: q input; dq input; ddq input; tau_control output; qd input; qd_dot input; qd_ddot input; force input; time input
function tau_control   = fcn(q, dq, ddq, qd, qd_dot, qd_ddot,force,...
                                                                  time)
% reset first qd_ddot
if (time < 0.003)
    qd_ddot = [0;0;0];
    qd_dot = [0;0;0];
    ddq = [0;0;0];
end


%% Joint Space variables

q1 = q(1);
q2 = q(2);
q3 = q(3);

dq1 = dq(1);
dq2 = dq(2);
dq3 = dq(3);

%% general physical parameters

l1 = 0.6731;
l2 = 0.432;
l3 = 0.434;
lc2 = 0.216;
lc3 = 0.164;
m2 = 15.46;
m3 = 9.55;
J = 0.302;

%% Inertia Matrix Parameters

J1 = m3 * lc3^2;
J12 = (m2 * lc2^2) + (m3 * l2^2);
J13 = l2 * lc3 * m3;


h11 = J + J1 * (sin(q2 + q3))^2 + J12 * (cos(q2))^2 + 2 * J13 * cos(q2) * sin(q2+q3);
h22 = J1 + J12 + 2 * J13 * sin(q3);
h23 = J1 + J13 * sin(q3);
h32 = h23;
h33 = J1;

H = [h11, 0 ,0 ;
    0 , h22, h23;
    0 , h32, h33];

%% Coriolis Matrix Parameters

c12_1 = J1 * sin(2 * (q1 + q2)) - J12 * sin(2 * q2) + 2 * J13 * cos(2 * q2 +q3);
c13_1 = J1 * sin(2 * (q2 + q3)) + 2 * J13 * cos(q2) * cos(q2 + q3);
c11_2 = (1/2) * (-J1 * sin(2 * (q2 + q3)) + J12 * sin(2 * q2) - 2 * J13 * cos(2 * q2 + q3));
c22_2 = 2 * J13 * cos(q3);
c23_2 = J13 * cos(q3);
c22_3 = -J13 * cos(q3) * dq2;
c11_3 = (-1/2) * (J1 * sin(2 * (q2 + q3)) + J13 * cos(q2) * cos(q2 + q3));

C = [0, c12_1 * dq1, c13_1 * dq3;
    c11_2 * dq1, 0 , c22_2 * dq2 + c23_2 * dq3;
    c11_3 * dq1, c22_3 * dq2, 0];

%% Vector of Potential Forces Parameters

g = 9.81;

g21 = -g * (lc3 * m3 * sin(q2 + q3) + lc2 * m2 * cos(q2) + l2 * m3 * cos(q2));
g31 = -g * (lc3 * m3 * sin(q2 + q3));

G = [0;
    g21;
    g31];


%% get Jacobians
J = jacobian(q);
dJ = dJacobian(q,dq);

%% convert to task space
Hp = inv(J') * H * inv(J);
Cp = inv(J') * C * inv(J) - Hp * dJ * inv(J);
Gp = inv(J') * G;

%% desired behaviour 
Hm = [1 0 0; 0 1 0; 0 0 1];
Dm = [20 0 0; 0 20 0; 0 0 20];
Km = [500 0 0; 0 500  0; 0 0 500];

%% get postion and its derivs
p = fwdKin(q);
dp = J * dq;
ddp = dJ * dq + J * ddq;

%% get desired postion and its derivs
pd = fwdKin(qd);
pd_dot = jacobian(qd) * qd_dot;
pd_ddot = dJacobian(qd,qd_dot) * qd_dot + jacobian(qd) * qd_ddot;

%% define u note

u_note = pd_ddot + inv(Hm) * (Dm * (pd_dot-dp) + Km*(pd - p) + force);
inv_hm = inv(Hm);
%% define tau_control

tau_control = J' * (Hp * u_note + Cp * dp + Gp - force);


function [X] = fwdKin(Q)
    s1 = sin(Q(1, :));
    c1 = cos(Q(1, :));
    s2 = sin(Q(2, :));
    c2 = cos(Q(2, :));
    s23 = sin(Q(2, :) + Q(3, :));
    c23 = cos(Q(2, :) + Q(3, :));
    l = [0.6731; 0.432; 0.434];
    
    X = zeros(3,1);
    X(1, :) = c1.*(l(2)*c2 + l(3)*s23);
    X(2, :) = s1.*(l(2)*c2 + l(3)*s23);
    X(3, :) = l(1) - l(2)*s2 + l(3)*c23;

function dJ = dJacobian(Q, dQ)
    l = [0.6731; 0.432; 0.434];
    s1 = sin(Q(1));
    c1 = cos(Q(1));
    s2 = sin(Q(2));
    c2 = cos(Q(2));
    s23 = sin(Q(2) + Q(3));
    c23 = cos(Q(2) + Q(3));

    % dJi derivative of each element of Jacobian wrt i-th variable            
    %--- 1 ---
    dJ1 = [-c1*(l(2)*c2 + l(3)*s23), -s1*(-l(2)*s2 + l(3)*c23), -l(3)*s1*c23;...
           -s1*(l(2)*c2 + l(3)*s23),  c1*(-l(2)*s2 + l(3)*c23),  l(3)*c1*c23;...
           0, 0, 0];
    %--- 2 ---   
    dJ2 = [-s1*(-l(2)*s2 + l(3)*c23), -c1*(l(2)*c2 + l(3)*s23), -l(3)*c1*s23;...
            c1*(-l(2)*s2 + l(3)*c23), -s1*(l(2)*c2 + l(3)*s23), -l(3)*s1*s23;...
            0, l(2)*s2 - l(3)*c23, -l(3)*c23];

    %--- 3 ---
    dJ3 = -l(3)*[ s1*c23, c1*s23, c1*s23;...
                 -c1*c23, s1*s23, s1*s23;...
                 0, c23, c23];
    %--- dJ ---
    dJ = dJ1*dQ(1) + dJ2*dQ(2) + dJ3*dQ(3);

function [J] = jacobian(q)

l = [0.6731; 0.432; 0.434];
s1 = sin(q(1));
c1 = cos(q(1));
s2 = sin(q(2));
c2 = cos(q(2));
s23 = sin(q(2) + q(3));
c23 = cos(q(2) + q(3));

J = zeros(3,3);

J(1, 1) = -s1*( l(2)*c2 + l(3)*s23);
J(1, 2) =  c1*(-l(2)*s2 + l(3)*c23);
J(1, 3) = l(3)*c1*c23;

J(2, 1) = c1*( l(2)*c2 + l(3)*s23);
J(2, 2) = s1*(-l(2)*s2 + l(3)*c23);
J(2, 3) = l(3)*s1*c23;

J(3, 2) = -l(2)*c2 - l(3)*s23;
J(3, 3) = -l(3)*s23;

== matlab function FinalProjectSimulation/Enabled and Triggered Subsystem2/If Action Subsystem/MATLAB Function ==
  data: q input; X output
function X = FWDKinematics(q)
%%% Forward Kinematic Function


%% Joint Space variables
% q is 3*1 vector of joint variables (radian), q = [q1;q2;q3]
q1 = q(1);
q2 = q(2);
q3 = q(3);

%% general physical parameters
l1 = 0.6731;
l2 = 0.432;
l3 = 0.434;
lc2 = 0.216;
lc3 = 0.164;

%% Forward Kinematic
% X is 3*1 vecto of end-effector position in task space, X = [x;y;z]

x = cos(q1) * (l2 * cos(q2) + l3 * sin(q2 + q3));
y = sin(q1) * (l2 * cos(q2) + l3 * sin(q2 + q3));
z = l1 - l2 * sin(q2) + l3 * cos(q2 + q3);

X = [x;y;z]

== matlab function FinalProjectSimulation/Enabled and Triggered Subsystem2/If Action Subsystem/Update Goal Point ==
  data: waypoints input; new_waypoints output; new_goal input
function new_waypoints = updateGoalPoint(waypoints,new_goal)
% updateGoalPoint 
%   update the goal point of the trajectory with a new goal that can change
%   with time.

new_waypoints = waypoints;
new_waypoints(:,end) = new_goal;

end
